simulink model "Highway_Lane_Detection_CS2018"  (R2014b)
settings: Solver=ode45  SolverMode=SingleTasking  StartTime=0  StopTime=12  FixedStep=0.001  RelTol=1e-3  AbsTol=1e-6
undefined symbols (not defined in the file): gray, Rec, SDTV, strel
libraries: visiontextngfix x6, Solver_SF x2, visionmorphops x2, visiontransforms x2, visionconversions x1, visionanalysis x1, visionstatistics x1, visionsinks x1
settings Model: CovSFcnEnable=on  ExtModeTrigMode=oneshot  ExtModeArmWhenConnect=off  Creator=ywata  LastModifiedBy=elowe
settings DataIOCC: LimitDataPoints=off  SignalLoggingSaveFormat=ModelDataLogs  SignalLoggingName=sigsOut
settings OptimizationCC: BlockReduction=off  BooleanDataType=off
settings DebuggingCC: SaveWithParameterizedLinksMsg=none  UnderspecifiedInitializationDetection=Classic  MergeDetectMultiDrivingBlocksExec=none  SignalResolutionControl=TryResolveAllWithWarning  SolverPrmCheckMsg=none  InheritedTsInSrcMsg=none  MultiTaskDSMMsg=warning  MultiTaskCondExecSysMsg=none  ParameterPrecisionLossMsg=none  FcnCallInpInsideContextMsg=EnableAllAsWarning  FrameProcessingCompatibilityMsg=error  StateNameClashWarn=warning
settings HardwareCC: TargetLongLongMode=on  TargetIntDivRoundTo=Zero  TargetEndianess=LittleEndian  TargetHWDeviceType=MATLAB Host  ProdEqTarget=off
settings RTWCC: TemplateMakefile=grt_vc.tmf
settings GRTTargetCC: TargetFcnLib=ansi_tfl_tmw.mat  GeneratePreprocessorConditionals=Use local settings  CombineOutputUpdateFcns=off  GRTInterface=on

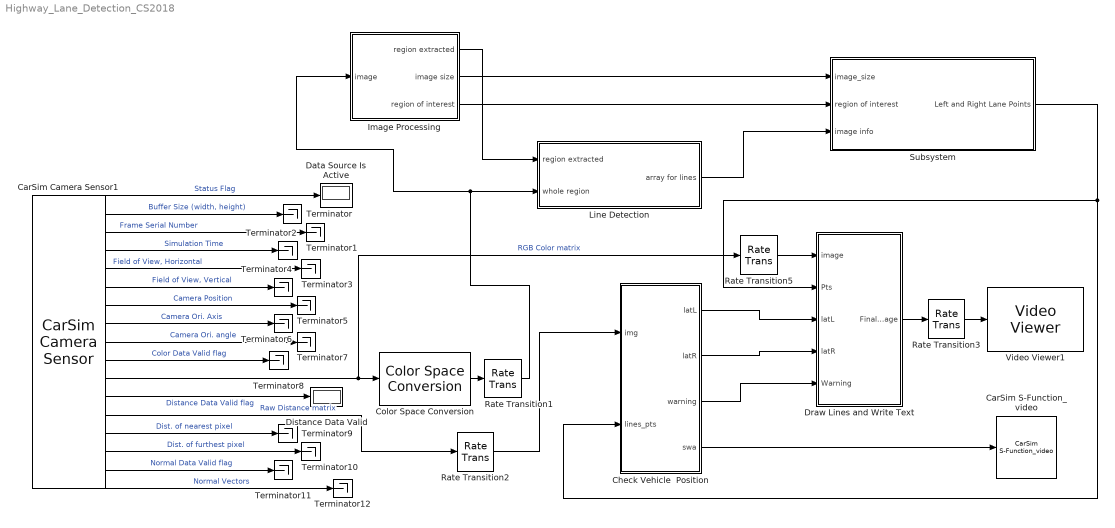
== system Highway_Lane_Detection_CS2018 ==
  CarSim Camera Sensor1 : Solver_SF/CarSim Camera Sensor  Priority=1
  CarSim S-Function_video : Solver_SF/CarSim S-Function_video  Priority=1  SIMFILE=simfile.sim
  Check Vehicle  Position : MATLAB Function  TreatAsAtomicUnit=on
  Color Space Conversion : visionconversions/Color Space  Conversion  conversion=Obsolete  conversionActive=R'G'B' to intensity  wp_str=D65  rec=Rec. 601 (SDTV)  sys=1125/60/2:1  imagePorts=One multidimensional signal
  Data Source Is Active : Display
  Distance Data Valid : Display
  Draw Lines and Write Text : Subsystem
  Image Processing : Subsystem
  "Line Detection " : Subsystem
  Rate Transition{1..3,5} (4 alike) : RateTransition  OutPortSampleTime=0.05
  Subsystem : Subsystem
  Terminator{,1..12} (13 alike) : Terminator
  Video Viewer1 : visionsinks/Video Viewer  inputType=Obsolete7b  imagePorts=One multidimensional signal  useColorMap=off  colormapValue=gray(256)  specRange=off  minInputVal=0  maxInputVal=255  FigPos=[1346 461 547 332]  AxisZoom=on  trueSizedOnce=off  OpenAtMdlStart=on  DefaultConfigurationName=vipscopes.VideoViewerScopeCfg
  wires:
  CarSim Camera Sensor1/11 -> Rate Transition5/1, Color Space Conversion/1  "RGB Color matrix"
  CarSim Camera Sensor1/1 -> Data Source Is Active/1  "Status Flag"
  CarSim Camera Sensor1/17 -> Terminator12/1  "Normal Vectors"
  CarSim Camera Sensor1/2 -> Terminator/1  "Buffer Size (width, height)"
  CarSim Camera Sensor1/14 -> Terminator9/1  "Dist. of nearest pixel"
  CarSim Camera Sensor1/15 -> Terminator10/1  "Dist. of furthest pixel"
  CarSim Camera Sensor1/16 -> Terminator11/1  "Normal Data Valid flag"
  CarSim Camera Sensor1/12 -> Distance Data Valid/1  "Distance Data Valid flag"
  CarSim Camera Sensor1/10 -> Terminator8/1  "Color Data Valid flag"
  CarSim Camera Sensor1/3 -> Terminator1/1  "Frame Serial Number"
  CarSim Camera Sensor1/4 -> Terminator2/1  "Simulation Time"
  CarSim Camera Sensor1/5 -> Terminator3/1  "Field of View, Horizontal"
  CarSim Camera Sensor1/6 -> Terminator4/1  "Field of View, Vertical"
  CarSim Camera Sensor1/7 -> Terminator5/1  "Camera Position"
  CarSim Camera Sensor1/8 -> Terminator6/1  "Camera Ori. Axis"
  CarSim Camera Sensor1/9 -> Terminator7/1  "Camera Ori. angle"
  Rate Transition1/1 -> Image Processing/1(image), "Line Detection "/2(whole region)
  Color Space Conversion/1 -> Rate Transition1/1
  CarSim Camera Sensor1/13 -> Rate Transition2/1  "Raw Distance matrix"
  Image Processing/1(region extracted) -> "Line Detection "/1(region extracted)
  Subsystem/1(Left and Right Lane Points) -> Draw Lines and Write Text/2(Pts), Check Vehicle  Position/2(lines_pts)
  Rate Transition2/1 -> Check Vehicle  Position/1(img)
  Check Vehicle  Position/4(swa) -> CarSim S-Function_video/1
  Image Processing/2(image size) -> Subsystem/1(image_size)
  Image Processing/3(region of interest) -> Subsystem/2(region of interest)
  "Line Detection "/1(array for lines) -> Subsystem/3(image info)
  Check Vehicle  Position/1(latL) -> Draw Lines and Write Text/3(latL)
  Check Vehicle  Position/2(latR) -> Draw Lines and Write Text/4(latR)
  Check Vehicle  Position/3(warning) -> Draw Lines and Write Text/5(Warning)
  Draw Lines and Write Text/1(Final Image) -> Rate Transition3/1
  Rate Transition3/1 -> Video Viewer1/1
  Rate Transition5/1 -> Draw Lines and Write Text/1(image)

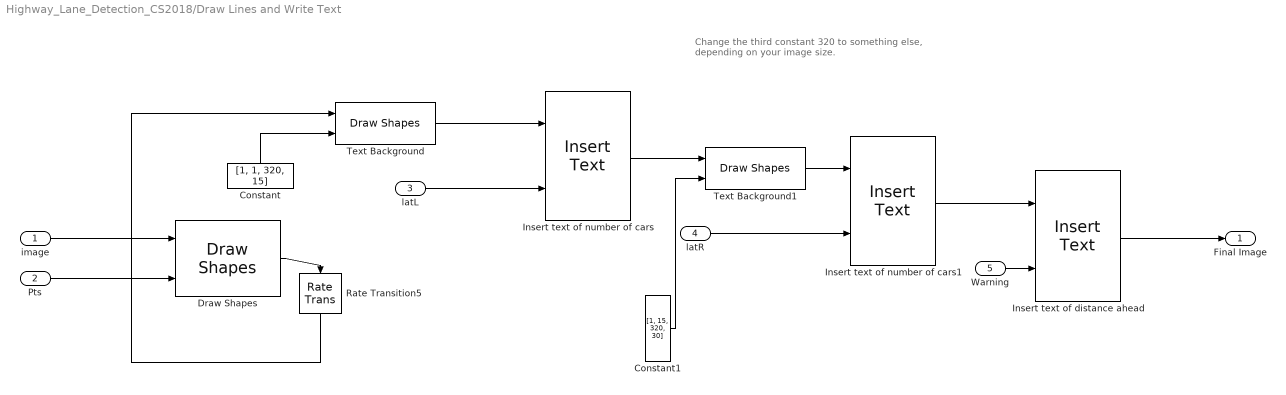
== system Highway_Lane_Detection_CS2018/Draw Lines and Write Text ==
  note: Change the third constant 320 to something else, depending on your image size.
  image : Inport
  Pts : Inport  Port=2
  latL : Inport  Port=3
  latR : Inport  Port=4
  Warning : Inport  Port=5
  Constant : Constant  Value=[1, 1, 320, 15]  OutDataTypeStr=uint32
  Constant1 : Constant  Value=[1, 15, 320, 30]  OutDataTypeStr=uint32
  Draw Shapes : visiontextngfix/Draw Shapes  shape=Lines  fill=off  lineWidth=5  fillClrSource=Specify via dialog  display=User-specified value  intensity=200  color=[200 255 100]  opacity=0.6  viewport=Entire image  antialiasing=off  inType=Obsolete  imagePorts=One multidimensional signal  prodOutputMode=Binary point scaling  prodOutputWordLength=32  prodOutputFracLength=14  memoryMode=Specify word length  memoryWordLength=16  memoryFracLength=14  roundingMode=Floor  overflowMode=off
  Insert text of distance ahead : visiontextngfix/Insert Text  inputType=Obsolete  theText={'','Drift to the Right', 'Drift to the Left'}  getTextLocFrom=Specify via dialog  textLoc=[160 100]  getTextColorFrom=Specify via dialog  textColor=[256 0 0]  getTextIntensityFrom=Specify via dialog  textIntensity=1  getTextOpacityFrom=Specify via dialog  textOpacity=1.0  dummyVar2=0  dummyVar3=0  dummyVar4=0  imagePorts=One multidimensional signal  isInputTransposed=off  fontFace=LucidaTypewriterRegular  dummyVar1=0  blockFontSize=14  antiAliased=off
  Insert text of number of cars : visiontextngfix/Insert Text  inputType=Obsolete  theText='Left Lateral Distance to the Line: %.1f m'  getTextLocFrom=Specify via dialog  textLoc=[5 1]  getTextColorFrom=Specify via dialog  textColor=[256 256 256]  getTextIntensityFrom=Specify via dialog  textIntensity=1  getTextOpacityFrom=Specify via dialog  textOpacity=1.0  dummyVar2=0  dummyVar3=0  dummyVar4=0  imagePorts=One multidimensional signal  isInputTransposed=off  fontFace=LucidaTypewriterRegular  dummyVar1=0  blockFontSize=12  antiAliased=on
  Insert text of number of cars1 : visiontextngfix/Insert Text  inputType=Obsolete  theText='Right Lateral Distance to the Line: %.1f m'  getTextLocFrom=Specify via dialog  textLoc=[5 25]  getTextColorFrom=Specify via dialog  textColor=[256 256 256]  getTextIntensityFrom=Specify via dialog  textIntensity=1  getTextOpacityFrom=Specify via dialog  textOpacity=1.0  dummyVar2=0  dummyVar3=0  dummyVar4=0  imagePorts=One multidimensional signal  isInputTransposed=off  fontFace=LucidaTypewriterRegular  dummyVar1=0  blockFontSize=12  antiAliased=on
  Rate Transition5 : RateTransition  OutPortSampleTime=0.05
  Text Background : visiontextngfix/Draw Shapes  shape=Rectangles  fill=on  lineWidth=1  fillClrSource=Specify via dialog  display=User-specified value  intensity=200  color=[0 0 0]  opacity=1  viewport=Entire image  antialiasing=off  inType=Obsolete  imagePorts=One multidimensional signal  prodOutputMode=Binary point scaling  prodOutputWordLength=32  prodOutputFracLength=14  memoryMode=Specify word length  memoryWordLength=16  memoryFracLength=14  roundingMode=Floor  overflowMode=off
  Text Background1 : visiontextngfix/Draw Shapes  shape=Rectangles  fill=on  lineWidth=1  fillClrSource=Specify via dialog  display=User-specified value  intensity=200  color=[0 0 0]  opacity=1  viewport=Entire image  antialiasing=off  inType=Obsolete  imagePorts=One multidimensional signal  prodOutputMode=Binary point scaling  prodOutputWordLength=32  prodOutputFracLength=14  memoryMode=Specify word length  memoryWordLength=16  memoryFracLength=14  roundingMode=Floor  overflowMode=off
  Final Image : Outport
  wires:
  Draw Shapes/1 -> Rate Transition5/1
  latL/1 -> Insert text of number of cars/2
  latR/1 -> Insert text of number of cars1/2
  Constant/1 -> Text Background/2
  Rate Transition5/1 -> Text Background/1
  Text Background/1 -> Insert text of number of cars/1
  Insert text of number of cars1/1 -> Insert text of distance ahead/1
  Insert text of number of cars/1 -> Text Background1/1
  Text Background1/1 -> Insert text of number of cars1/1
  Constant1/1 -> Text Background1/2
  Warning/1 -> Insert text of distance ahead/2
  image/1 -> Draw Shapes/1
  Pts/1 -> Draw Shapes/2
  Insert text of distance ahead/1 -> Final Image/1

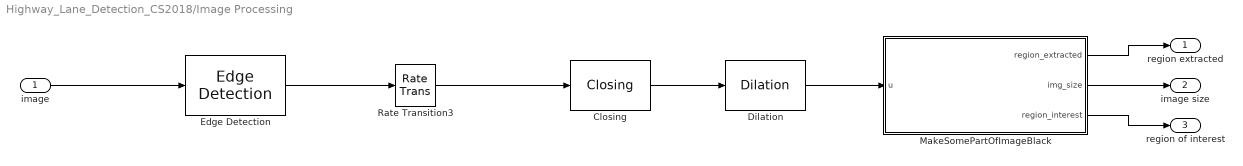
== system Highway_Lane_Detection_CS2018/Image Processing ==
  image : Inport
  Closing : visionmorphops/Closing  nhoodsrc=Specify via dialog  strel=strel('line',5,45)
  Dilation : visionmorphops/Dilation  nhoodsrc=Specify via dialog  strel=[1 1; 1 1]
  Edge Detection : visionanalysis/Edge Detection  method=Sobel  outputType=Binary image  userDefinedThreshold=on  thresholdSource=Specify via dialog  threshold=30  thresholdTuning=4  edgeThinning=off  threshold_canny=[0.25 0.60]  autoPercent=70  sigma=1  prodOutputMode=Binary point scaling  prodOutputWordLength=32  prodOutputFracLength=8  roundingMode=Floor  overflowMode=off
  MakeSomePartOfImageBlack : MATLAB Function  TreatAsAtomicUnit=on
  Rate Transition3 : RateTransition  OutPortSampleTime=0.05
  region extracted : Outport
  image size : Outport  Port=2
  region of interest : Outport  Port=3
  wires:
  Edge Detection/1 -> Rate Transition3/1
  Rate Transition3/1 -> Closing/1
  Dilation/1 -> MakeSomePartOfImageBlack/1(u)
  Closing/1 -> Dilation/1
  image/1 -> Edge Detection/1
  MakeSomePartOfImageBlack/1(region_extracted) -> region extracted/1
  MakeSomePartOfImageBlack/2(img_size) -> image size/1
  MakeSomePartOfImageBlack/3(region_interest) -> region of interest/1

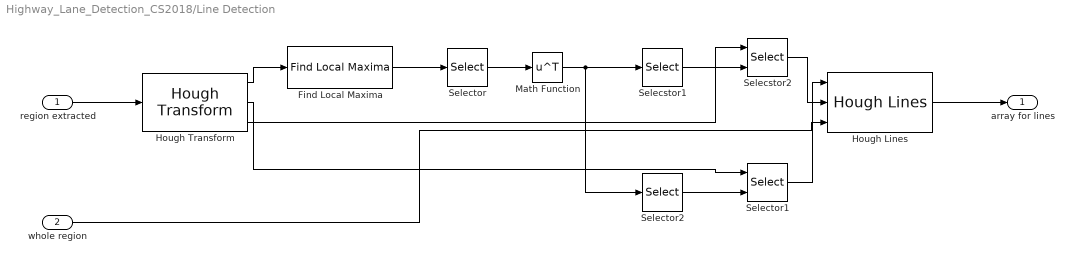
== system Highway_Lane_Detection_CS2018/Line Detection  ==
  region extracted : Inport
  whole region : Inport  Port=2
  Find Local Maxima : visionstatistics/Find Local Maxima  num_peaks=20  nhood_size=[3 3]  src_thresh=Obsolete9b  src_thresh_inuse=Specify via dialog  threshold=30  inputIsHough=on  dt_peak=uint32  isOutVarDim=on  dt_count=uint32
  Hough Lines : visiontransforms/Hough Lines  sineCompMethod=Trigonometric function  thetaRes=pi/180  firstCoeffMode=Specify word length  firstCoeffWordLength=16  firstCoeffFracLength=15  prodOutputMode=Binary point scaling  prodOutputWordLength=32  prodOutputFracLength=16  roundingMode=Nearest  overflowMode=on
  Hough Transform : visiontransforms/Hough Transform  theta_res=pi/30  rho_res=1  out_theta_rho=on  outdtmode=double  firstCoeffMode=Binary point scaling  firstCoeffWordLength=16  firstCoeffFracLength=14  secondCoeffMode=Binary point scaling  secondCoeffWordLength=32  secondCoeffFracLength=16  outputMode=Binary point scaling  outputWordLength=16  outputFracLength=0  accumMode=Binary point scaling  accumWordLength=32  accumFracLength=20  prodOutputMode=Binary point scaling  prodOutputWordLength=32  prodOutputFracLength=20  memoryMode=Binary point scaling  memoryWordLength=32  memoryFracLength=16  roundingMode=Nearest  overflowMode=on
  Math Function : Math  Operator=transpose  SaturateOnIntegerOverflow=on
  Selecstor1 : Selector  NumberOfDimensions=2  InputPortWidth=2  IndexOptions=Index vector (dialog),Select all  Indices=1,[2 1]  OutputSizes=1,1
  Selecstor2 : Selector  NumberOfDimensions=2  InputPortWidth=2  IndexOptions=Select all,Index vector (port)  Indices=1,[2 1]  OutputSizes=1,1
  Selector : Selector  NumberOfDimensions=2  InputPortWidth=2  IndexOptions=Select all,Index vector (dialog)  Indices=[1 3],[2 1]  OutputSizes=1,1
  Selector1 : Selector  NumberOfDimensions=2  InputPortWidth=2  IndexOptions=Select all,Index vector (port)  Indices=2,[2 1]  OutputSizes=1,1
  Selector2 : Selector  NumberOfDimensions=2  InputPortWidth=2  IndexOptions=Index vector (dialog),Select all  Indices=2,[2 1]  OutputSizes=1,1
  array for lines : Outport
  wires:
  whole region/1 -> Hough Lines/3
  Hough Transform/1 -> Find Local Maxima/1
  Find Local Maxima/1 -> Selector/1
  Selector/1 -> Math Function/1
  Math Function/1 -> Selector2/1, Selecstor1/1
  Hough Transform/3 -> Selecstor2/1
  Selecstor1/1 -> Selecstor2/2
  Selector2/1 -> Selector1/2
  Hough Transform/2 -> Selector1/1
  Selecstor2/1 -> Hough Lines/2
  Selector1/1 -> Hough Lines/1
  Hough Lines/1 -> array for lines/1
  region extracted/1 -> Hough Transform/1

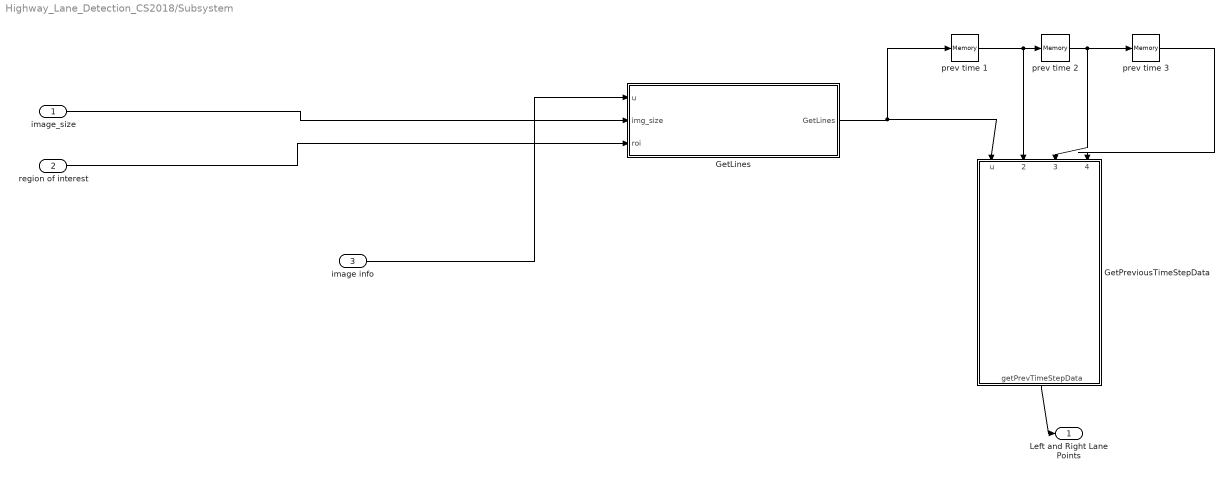
== system Highway_Lane_Detection_CS2018/Subsystem ==
  image_size : Inport
  region of interest : Inport  Port=2
  image info : Inport  Port=3
  GetLines : MATLAB Function  TreatAsAtomicUnit=on
  GetPreviousTimeStepData : MATLAB Function  TreatAsAtomicUnit=on
  "prev time 1 " : Memory
  prev time 2 : Memory
  prev time 3 : Memory
  Left and Right Lane Points : Outport
  wires:
  image_size/1 -> GetLines/2(img_size)
  region of interest/1 -> GetLines/3(roi)
  GetLines/1(GetLines) -> "prev time 1 "/1, GetPreviousTimeStepData/1(u)
  prev time 2/1 -> prev time 3/1, GetPreviousTimeStepData/3(prev_time2)
  prev time 3/1 -> GetPreviousTimeStepData/4(prev_time3)
  image info/1 -> GetLines/1(u)
  "prev time 1 "/1 -> GetPreviousTimeStepData/2(prev_time1), prev time 2/1
  GetPreviousTimeStepData/1(getPrevTimeStepData) -> Left and Right Lane Points/1

== matlab function Highway_Lane_Detection_CS2018/Subsystem/GetLines ==
  data: u input size=20 4; GetLines output size=2 4; img_size input; roi input
function GetLines= fcn(u, img_size, roi)

[m, n] = size(u);

% make the varaible length array to fixed length, 20 x 4
m_fixed = 20;
n_fixed = 4;

u1 = zeros(m_fixed,n_fixed);
for i=1:m
    for j=1:n
        u1(i,j)=u(i,j);
    end
end
right_array = zeros(m_fixed,n_fixed, 'int32');
left_array = zeros(m_fixed,n_fixed, 'int32');

i = 1;  % right_array counter
j = 1;  % left_array counter

for  x = 1:m
    if (u1(x,1) == u1(x,3))
        if (u1(x,2) ~= 0)
            t1 = 1;
        end
    end
    if u1(x,3) > img_size(2)/2 % column = 320/2
        if (u1(x,1) ~= u1(x,3)) & (u1(x,2) ~= u1(x,4))
            right_array(i,:) = u1(x,:);
            i = i + 1;
        end
    else
        if (u1(x,1) ~= u1(x,3)) & (u1(x,2) ~= u1(x,4))
            left_array(j,:) = u1(x,:);
            j = j + 1;
        end
    end
end

new_left_array = left_array(any(left_array~=0,2),:);
if isempty(new_left_array)
    new_left_array = zeros(1,4, 'int32');
end
new_right_array = right_array(any(right_array~=0,2),:);
if isempty(new_right_array)
    new_right_array = zeros(1,4, 'int32');
end

[m1, n1] = size(new_left_array);
[m2, n2] = size(new_right_array);
if (m1 == 1)
    left_average = new_left_array;
else
    left_average = int32(mean(new_left_array));
end
if (m2 == 1)
    right_average = new_right_array;
else
    right_average = int32(mean(new_right_array));
end

upper_bound = roi(2);
if (all(left_average(1,:)) ~= 0)
    left_upper_pts = (left_average(1)-left_average(3))*(upper_bound-left_average(4))...
    /(left_average(2)-left_average(4)) + left_average(3);
    left_average = [left_upper_pts, upper_bound, left_average(3), left_average(4)];
end
left_average = int32(left_average);

if (all(right_average(1,:)) ~= 0)
    right_upper_pts = (right_average(1)-right_average(3))*(upper_bound-right_average(4))...
    /(right_average(2)-right_average(4)) + right_average(3);
    right_average = [right_upper_pts, upper_bound, right_average(3), right_average(4)];
end
right_average = int32(right_average);

% don't want to draw the line from the top to bottom.
% calculate somewhere 1/3 from the bottom. (i.e., 2/3 from the top)
%print left_average, left_average
 
%GetLines = cat(1, left_average, right_average);
GetLines = zeros(2,4, 'int32');
for i=1:4
  GetLines(1,i) = left_average(1,i);
  GetLines(2,i) = right_average(1,i);
end

if (GetLines(1,1) == GetLines(1,3))
    t1 = 0;
end

== matlab function Highway_Lane_Detection_CS2018/Check Vehicle  Position ==
  data: img input; latL output; lines_pts input; latR output; warning output int32; swa output
function [latL, latR, warning, swa] = lateral_detection(img,lines_pts)

[row, col] = size(img);
left_line_dist = single(0.0);
right_line_dist = single(0.0);
lat_on_pixel_L = 0;
lat_on_pixel_R = col;
ang_to_left_lane = 0;
ang_to_right_lane = 0;
latL = single(0.0);
latR = single(0.0);
warning = int32(1);
swa = 5;

angle_to_vehicle = 90.0;
% assuming the field view is 55.  If not, change here.
fov = 55.0;
% size of img => [row, column] = [200 320] for this example
% lines_pts = [upper_col, upper_row, lower_col, lower_col]
if all(lines_pts(1,:) ~= 0)
    left_line_dist = img(lines_pts(1,2), lines_pts(1,1));
    lat_on_pixel_L = col/2 - lines_pts(1,1);
    ang_to_left_lane = single(lat_on_pixel_L*27.5/160);
    latL = left_line_dist*tan(ang_to_left_lane/180*pi);
end

if all(lines_pts(2,:) ~= 0)
    right_line_dist = img(lines_pts(2,2), lines_pts(2,1));
    lat_on_pixel_R = col/2 - lines_pts(2,1);
    ang_to_right_lane = single(lat_on_pixel_R*27.5/160);
    latR = right_line_dist*tan(ang_to_right_lane/180*pi);
end

%{'','Drift to the Right', 'Drift to the Left'}
if (latR ~= 0 & latL ~= 0)
    if abs(abs(latL) - abs(latR)) > 0.7
        if abs(latL) > abs(latR)
            warning = int32(2);
            swa = 25.0;
        else
            warning = int32(3);
            swa = -25.0;
        end
    end
end
if (abs(latR) < 1.0 & latR ~= 0)
    warning = int32(2);
    swa = 25.0;
end
if (abs(latL) < 1.0 & latL ~= 0)
    warning = int32(3);
    swa = -25.0;
end

== matlab function Highway_Lane_Detection_CS2018/Image Processing/MakeSomePartOfImageBlack ==
  data: u input; region_extracted output; img_size output; region_interest output
function [region_extracted, img_size, region_interest]= MakeSomePartBlack(u)

[rows, columns]  = size(u);
c = zeros(rows, columns);

img_size = [rows, columns];
half_rows = rows/2;
half_columns = columns/2;

two_third_from_top = int32((2*rows)/3);

region_interest = [0, two_third_from_top, columns, rows-two_third_from_top];

% use the following for linear fit.  start with 10 points of x, y pairs.
pts_dim = 10;
left_pts = int32([]);
coder.varsize('left_pts', [10*columns, 2]);
right_pts = [];
row_region = int32(rows*3/5);
rows_in = row_region;
spacing = int32((rows-row_region)/9);
% remove the horizon.  ROI is the 2/5 bottom.
for  x = 1:rows
  for y = 1:columns
      if x < row_region;
        c(x,y) = 0;
      else
          if y <= half_columns
              if x < -(half_rows/half_columns)*y + rows
              %if x < -(half_rows/half_columns)*y + rows*3/4
                  c(x,y) = 0;
              else
                  c(x,y) = u(x,y);
              end                  
          else
              if x < (half_rows/half_columns)*y
              %if x < ((half_rows/2)/half_columns)*y
                  c(x,y) = 0;
              else
                  c(x,y) = u(x,y);
              end
          end
      end
  end
end


region_extracted = logical(c);

== matlab function Highway_Lane_Detection_CS2018/Subsystem/GetPreviousTimeStepData ==
  data: u input; getPrevTimeStepData output; prev_time1 input; prev_time2 input; prev_time3 input
function getPrevTimeStepData= fcn(u, prev_time1, prev_time2, prev_time3)

getPrevTimeStepData= u;
if all(u(1,:) == 0)
    prev_time_r = prev_time1(1,:);
    if (all(prev_time1(1,:)) == 0)
        if (all(prev_time2(1,:)) == 0)
            prev_time_r = prev_time3(1,:);
        else
            prev_time_r = prev_time2(1,:);
        end
    end
    getPrevTimeStepData(1,:) = prev_time_r;
end
if all(u(2,:) == 0)
    prev_time_l = prev_time1(1,:);
    if (all(prev_time1(2,:)) == 0)
        if (all(prev_time2(2,:)) == 0)
            prev_time_l = prev_time3(2,:);
        else
            prev_time_l = prev_time2(2,:);
        end
    end
    getPrevTimeStepData(2,:) = prev_time_l;
end
